simulink model "total_system"  (R2025b)
settings: Solver=FixedStepAuto  StartTime=0.0  StopTime=25  FixedStep=Ts  RelTol=1e-3
values from neighbouring files (symbols this model uses):
  poles = 2    [constants.m]
settings Model: TunableVars=J_AD,J_ICE,M_AD_nom,P_ballast_nom,P_oil_max,P_oil_min,T_AD_max,T_amb,T_ballast_max,T_cool_max,a_const,ad_fun_acceleration,b_const,k_heat,k_loss,k_loss0,k_rad_AD,k_rad_ballast,k_radiator,omega_ICE_max_prir,omega_ICE_max_run,tau,tau_AD_base,tau_ballast,tau_cool  TunableVarsStorageClass=Auto,Auto,Auto,Auto,Auto,Auto,Auto,Auto,Auto,Auto,Auto,Auto,Auto,Auto,Auto,Auto,Auto,Auto,Auto,Auto,Auto,Auto,Auto,Auto,Auto  TunableVarsTypeQualifier=,,,,,,,,,,,,,,,,,,,,,,,,  Creator=user  LastModifiedBy=user
settings OptimizationCC: DefaultParameterBehavior=Inlined  UseDivisionForNetSlopeComputation=on  GainParamInheritBuiltInType=on  UseFloatMulNetSlope=on  StrengthReduction=on  PassReuseOutputArgsAs=Individual arguments  ZeroExternalMemoryAtStartup=off  ZeroInternalMemoryAtStartup=off  NoFixptDivByZeroProtection=on  EfficientFloat2IntCast=on  OptimizeBlockOrder=speed  OptimizationPriority=Speed  OptimizationCustomize=off  MultiThreadedLoops=on  AutoScheduleForLoops=on  EfficientTunableParamExpr=on
settings DebuggingCC: ParameterTunabilityLossMsg=error
settings HardwareCC: ProdBitPerLong=64.0  ProdLongLongMode=on  ProdHWDeviceType=Intel->x86-64 (Linux 64)
settings SFSimCC: MATLABDynamicMemAlloc=off  SimTargetLang=C++  SimDLTargetLibrary=mkl-dnn
settings RTWCC: SystemTargetFile=ert.tlc  GenCodeOnly=on  TemplateMakefile=ert_default_tmf  GenerateReport=on  BuildConfiguration=Faster Runs  LaunchReport=on  TargetLang=C++  Description=Embedded Coder
settings CodeAppCC: ForceParamTrailComments=on  IgnoreCustomStorageClasses=off  OperatorAnnotations=on  SimulinkDataObjDesc=on  SFDataObjDesc=on  CustomSymbolStrGlobalVar=rt$N$M  CustomSymbolStrType=$N$M  CustomSymbolStrFcn=$N$M$F  CustomSymbolStrMacro=$N$M  InsertBlockDesc=on
settings ERTTargetCC: InlinedParameterPlacement=Hierarchical  RootIOFormat=Structure reference  ERTCustomFileTemplate=example_file_process.tlc  TargetLangStandard=C++17 (ISO)  GenerateSampleERTMain=on  CodeInterfacePackaging=C++ class  SubcomponentCodeInterfacePackaging=C++ class  SupportContinuousTime=on

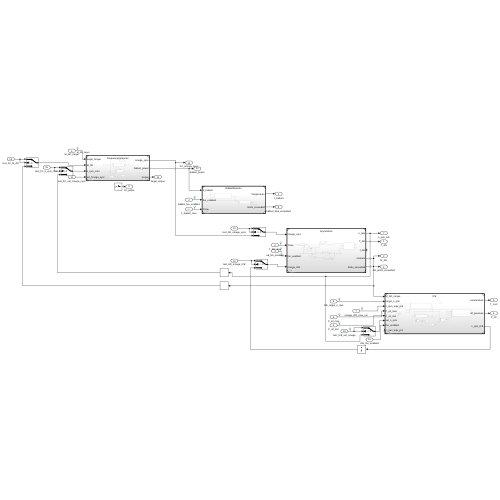
[thumbnail: Simulink's stored preview of the top-level diagram]
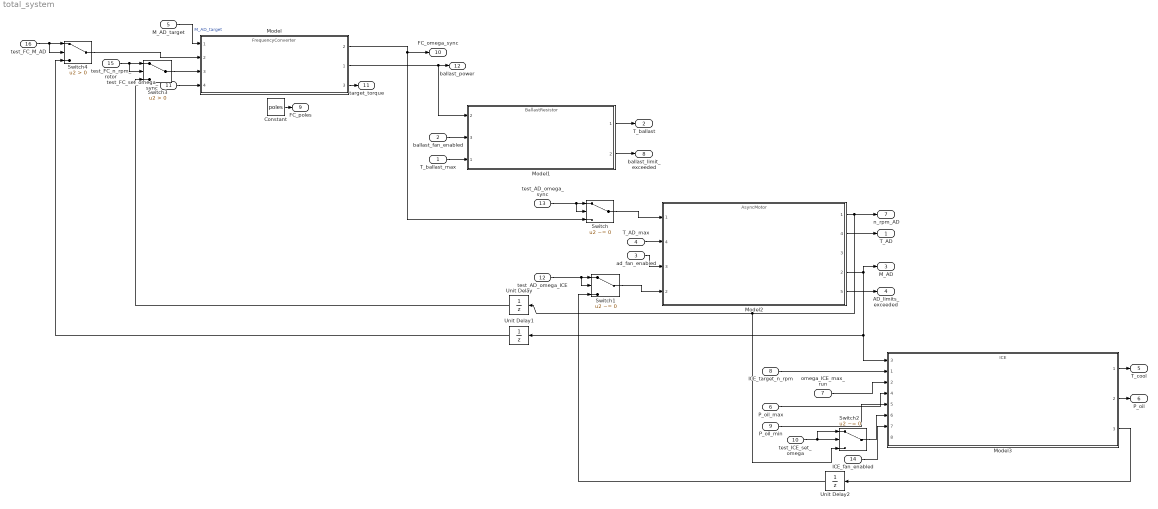
== system total_system ==
  T_ballast_max : Inport
  ballast_fan_enabled : Inport  Port=2
  ad_fan_enabled : Inport  Port=3
  T_AD_max : Inport  Port=4
  M_AD_target : Inport  Port=5
  P_oil_max : Inport  Port=6
  omega_ICE_max_run : Inport  Port=7
  ICE_target_n_rpm : Inport  Port=8
  P_oil_min : Inport  Port=9
  test_ICE_set_omega : Inport  Port=10
  test_FC_set_omega_sync : Inport  Port=11
  test_AD_omega_ICE : Inport  Port=12
  test_AD_omega_sync : Inport  Port=13
  ICE_fan_enabled : Inport  Port=14
  test_FC_n_rpm_rotor : Inport  Port=15
  test_FC_M_AD : Inport  Port=16
  Constant : Constant  Value=poles
  Model : ModelReference  ModelNameDialog=FrequencyConverter.slx  SimulationMode=Normal  ModelReferenceVersion=1.267
      settings: PortSchema="{\"entries\":[{\"content\":{\"sides\":[{\"content\":{\"connectorIds\":[\"In1\",\"In2\",\"In3\",\"In4\"]},\"type\":\"ConnectorPlacement.EquallySpacedRectSide\",\"uuid\":\"fb7b68ac-eebb-4afa-a640-f8ee29b918e7\"},{\"content\":{\"connectorIds\":[\"Out2\",\"Out1\",\"Out3\"],\"side\":\"RIGHT\"},\"type\":\"ConnectorPlacement.EquallySpacedRectSide\",\"uuid\":\"36a7af26-9da5-47de-83be-fc5a8e1e3567\"},{\"content\":{\"side\":\"TOP\"},\"type\":\"ConnectorPlacement.EquallySpacedRectSide\",\"uuid\":\"14735526-1400-48e1-8893-8e3db4005e87\"}]},\"type\":\"ConnectorPlacement.EquallySpacedConnector\",\"uuid\":\"3f09416c-462b-48b5-8071-b535eef128e8\"}],\"packageUris\":[\"http://schema.mathworks.com/mf0/Connector/R2020b\"],\"version\":\"1.0\"}"
  Model1 : ModelReference  ModelNameDialog=BallastResistor.slx  SimulationMode=Normal  ModelReferenceVersion=1.239
      settings: PortSchema="{\"entries\":[{\"content\":{\"sides\":[{\"content\":{\"connectorIds\":[\"In2\",\"In3\",\"In1\"]},\"type\":\"ConnectorPlacement.EquallySpacedRectSide\",\"uuid\":\"7f109583-06ea-4128-9ee5-b1f60cf269dc\"},{\"content\":{\"connectorIds\":[\"Out1\",\"Out2\"],\"side\":\"RIGHT\"},\"type\":\"ConnectorPlacement.EquallySpacedRectSide\",\"uuid\":\"3ed18453-e43c-4600-8919-fb5fb0e1ce83\"},{\"content\":{\"side\":\"TOP\"},\"type\":\"ConnectorPlacement.EquallySpacedRectSide\",\"uuid\":\"5bef5430-3b3c-4fa1-bb01-31f9fd9d9302\"}]},\"type\":\"ConnectorPlacement.EquallySpacedConnector\",\"uuid\":\"126d711d-4c62-4e17-b781-2a3b986b6ad3\"}],\"packageUris\":[\"http://schema.mathworks.com/mf0/Connector/R2020b\"],\"version\":\"1.0\"}"
  Model2 : ModelReference  ModelNameDialog=AsyncMotor.slx  SimulationMode=Normal  ModelReferenceVersion=1.349
      settings: PortSchema="{\"entries\":[{\"content\":{\"sides\":[{\"content\":{\"connectorIds\":[\"In1\",\"In4\",\"In3\",\"In2\"]},\"type\":\"ConnectorPlacement.EquallySpacedRectSide\",\"uuid\":\"5b7a86e2-c3ef-4dc3-8fb2-3083449b5a6f\"},{\"content\":{\"connectorIds\":[\"Out1\",\"Out4\",\"Out3\",\"Out2\",\"Out5\"],\"side\":\"RIGHT\"},\"type\":\"ConnectorPlacement.EquallySpacedRectSide\",\"uuid\":\"3c7dfd5a-510a-493e-8b1f-04656407d19e\"},{\"content\":{\"side\":\"TOP\"},\"type\":\"ConnectorPlacement.EquallySpacedRectSide\",\"uuid\":\"215599f8-0360-463d-8322-4f13a94e0c21\"}]},\"type\":\"ConnectorPlacement.EquallySpacedConnector\",\"uuid\":\"e1896410-dac0-4be5-a85a-2de1e90a7d9b\"}],\"packageUris\":[\"http://schema.mathworks.com/mf0/Connector/R2020b\"],\"version\":\"1.0\"}"
  Model3 : ModelReference  ModelNameDialog=ICE.slx  SimulationMode=Normal  ModelReferenceVersion=1.460
      settings: PortSchema="{\"entries\":[{\"content\":{\"sides\":[{\"content\":{\"connectorIds\":[\"In3\",\"In1\",\"In2\",\"In4\",\"In5\",\"In6\",\"In7\",\"In8\"]},\"type\":\"ConnectorPlacement.EquallySpacedRectSide\",\"uuid\":\"03a90139-1e88-4267-b314-cfb62ce18d1a\"},{\"content\":{\"connectorIds\":[\"Out1\",\"Out2\",\"Out3\"],\"side\":\"RIGHT\"},\"type\":\"ConnectorPlacement.EquallySpacedRectSide\",\"uuid\":\"8d42cf4f-92cc-4bcf-ab8f-3d0b14eeba6d\"},{\"content\":{\"side\":\"TOP\"},\"type\":\"ConnectorPlacement.EquallySpacedRectSide\",\"uuid\":\"ec99585d-049d-4d71-a81c-ffb7baa0e97b\"}]},\"type\":\"ConnectorPlacement.EquallySpacedConnector\",\"uuid\":\"e88772a1-3eed-4319-bd37-78f8632c8d7a\"}],\"packageUris\":[\"http://schema.mathworks.com/mf0/Connector/R2020b\"],\"version\":\"1.0\"}"
  Switch : Switch  Criteria=u2 ~= 0  SaturateOnIntegerOverflow=off  InputSameDT=off
  Switch1 : Switch  Criteria=u2 ~= 0  SaturateOnIntegerOverflow=off  InputSameDT=off
  Switch2 : Switch  Criteria=u2 ~= 0  SaturateOnIntegerOverflow=off  InputSameDT=off
  Switch3 : Switch  Criteria=u2 > Threshold  SaturateOnIntegerOverflow=off  InputSameDT=off
  Switch4 : Switch  Criteria=u2 > Threshold  SaturateOnIntegerOverflow=off  InputSameDT=off
  Unit Delay : UnitDelay  SampleTime=-1  HasFrameUpgradeWarning=on
  Unit Delay1 : UnitDelay  SampleTime=-1  HasFrameUpgradeWarning=on
  Unit Delay2 : UnitDelay  SampleTime=-1  HasFrameUpgradeWarning=on
  T_AD : Outport
  T_ballast : Outport  Port=2
  M_AD : Outport  Port=3
  AD_limits_exceeded : Outport  Port=4
  T_cool : Outport  Port=5
  P_oil : Outport  Port=6
  n_rpm_AD : Outport  Port=7
  ballast_limit_exceeded : Outport  Port=8
  FC_poles : Outport  Port=9
  FC_omega_sync : Outport  Port=10
  target_torque : Outport  Port=11
  ballast_power : Outport  Port=12
  wires:
  Model1/1 -> T_ballast/1
  ballast_fan_enabled/1 -> Model1/3
  T_ballast_max/1 -> Model1/1
  Unit Delay/1 -> Switch3/3
  Unit Delay1/1 -> Switch4/3
  M_AD_target/1 -> Model/1  "M_AD_target"
  Model3/3 -> Unit Delay2/1
  Model3/1 -> T_cool/1
  Model3/2 -> P_oil/1
  P_oil_max/1 -> Model3/4
  omega_ICE_max_run/1 -> Model3/2
  ICE_target_n_rpm/1 -> Model3/1
  P_oil_min/1 -> Model3/5
  test_FC_set_omega_sync/1 -> Model/4
  Model2/2 -> M_AD/1, Unit Delay1/1, Model3/3
  Model2/1 -> n_rpm_AD/1, Unit Delay/1, Switch2/3
  Model/1 -> ballast_power/1, Model1/2
  Unit Delay2/1 -> Switch1/3
  Model/2 -> FC_omega_sync/1, Switch/3
  Switch/1 -> Model2/1
  test_ICE_set_omega/1 -> Switch2/2, Switch2/1
  Switch2/1 -> Model3/6
  test_AD_omega_sync/1 -> Switch/2, Switch/1
  test_AD_omega_ICE/1 -> Switch1/2, Switch1/1
  ICE_fan_enabled/1 -> Model3/7
  Model1/2 -> ballast_limit_exceeded/1
  Model2/4 -> T_AD/1
  Model2/5 -> AD_limits_exceeded/1
  T_AD_max/1 -> Model2/4
  ad_fan_enabled/1 -> Model2/3
  Switch1/1 -> Model2/2
  Constant/1 -> FC_poles/1
  Model/3 -> target_torque/1
  test_FC_n_rpm_rotor/1 -> Switch3/2, Switch3/1
  Switch3/1 -> Model/3
  test_FC_M_AD/1 -> Switch4/2, Switch4/1
  Switch4/1 -> Model/2
